simulink model "Adaptive_7DOF"  (R2024a)
settings: Solver=ode4  StartTime=0.0  StopTime=20  FixedStep=0.01  RelTol=1e-3
model workspace (MAT data in the model file):
  e2 = Simulink.Signal
  e2.DataType = 'auto'
  e2.Dimensions = [4 1]
  e2.DimensionsMode = 'Fixed'
  e2.Complexity = 'auto'
  e2.SampleTime = -1
  e2.SamplingMode = 'auto'
libraries: aerolibconvert2 x20
settings Model: Creator=hp  LastModifiedBy=somesh
settings SolverCC: ZeroCrossAlgorithm=Adaptive
settings DataIOCC: ReturnWorkspaceOutputs=off
settings DebuggingCC: IgnoredZcDiagnostic=none  UnderSpecifiedDimensionMsg=warning
settings RTWCC: GPUComputeCapability=3.5

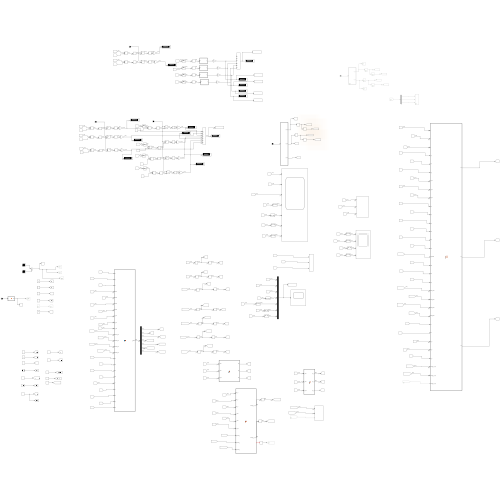
[thumbnail: Simulink's stored preview of the top-level diagram]
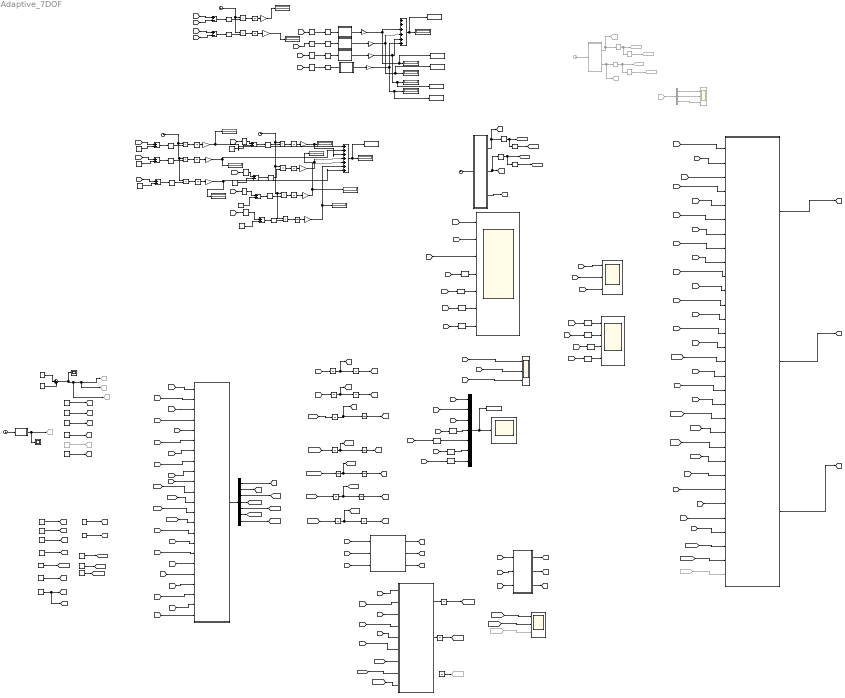
== system Adaptive_7DOF ==
  Abs{,1..12} (13 alike) : Abs  SaturateOnIntegerOverflow=off
  Angle Conversion{,1..19} (20 alike) : aerolibconvert2/Angle Conversion  IU=rad  OU=deg
  Clock{,1,5,7..8} (5 alike) : Clock
  Clock2 : Clock  Commented=on
  Constant : Constant  Value=6.1
  Constant1 : Constant  Value=15.6
  Constant10 : Constant  Value=14.77
  Constant11 : Constant  Value=0.5
  Constant12 : Constant  Value=0.6
  Constant13 : Constant  Value=32.11
  Constant14 : Constant  Value=30
  Constant15 : Constant  Value=17.55
  Constant{3,8,16..17} (4 alike) : Constant
  Constant18 : Constant  Value=29.41
  Constant19 : Constant  Value=43.34
  Constant2 : Constant  Value=2
  Constant20 : Constant  Value=1.5
  Constant21 : Constant  Value=0.01
  Constant22 : Constant  Value=0.005
  Constant4 : Constant  Commented=on  Value=0.5
  Constant{6..7,48..49} (4 alike) : Constant  Value=0
  Constant5 : Constant  Value=0.5
  Constant9 : Constant  Value=0.7
  Demux : Demux  Outputs=7
  Demux3 : Demux  Commented=on  Outputs=3
  Derivative{,1..3} (4 alike) : Derivative
  Derivative{4..7} (4 alike) : Derivative  Commented=on
  Display{1..4,25,28..29,39,53..59} (15 alike) : Display
  From110 : From  Commented=on  GotoTag=omega_z_cap
  From170 : From  Commented=on  GotoTag=qx_d
  From98 : From  Commented=on  GotoTag=omega_z_cap
  Gain{,1..12} (13 alike) : Gain
  Goto18 : Goto  Commented=on  GotoTag=Fx
  Goto19 : Goto  Commented=on  GotoTag=Fy
  Goto24 : Goto  Commented=on  GotoTag=l1
  Goto49 : Goto  Commented=on  GotoTag=qs_d
  Goto51 : Goto  Commented=on  GotoTag=qx_d
  Goto52 : Goto  Commented=on  GotoTag=Fz
  Goto53 : Goto  Commented=on  GotoTag=qs_d_Dot
  Goto54 : Goto  Commented=on  GotoTag=qs_d_DDot
  Goto55 : Goto  Commented=on  GotoTag=qx_d_Dot
  Goto56 : Goto  Commented=on  GotoTag=qx_d_DDot
  Goto61 : Goto  Commented=on  GotoTag=m2
  Goto64 : Goto  Commented=on  GotoTag=omega_z_cap
  Integrator{,1..7,12..20,22..25} (21 alike) : Integrator
  Integrator{8..11} (4 alike) : Integrator  WrapState=on  WrappedStateUpperValue=pi/2  WrappedStateLowerValue=-pi/2
  Integrator21 : Integrator  InitialCondition=0.5
  MATLAB Function : MATLAB Function  TreatAsAtomicUnit=on
  MATLAB Function1 : MATLAB Function  TreatAsAtomicUnit=on
  MATLAB Function13 : MATLAB Function  TreatAsAtomicUnit=on
  MATLAB Function16 : MATLAB Function  TreatAsAtomicUnit=on
  MATLAB Function2 : MATLAB Function  TreatAsAtomicUnit=on
  MATLAB Function20 : MATLAB Function  TreatAsAtomicUnit=on
  MATLAB Function3 : MATLAB Function  TreatAsAtomicUnit=on
  MATLAB Function4 : MATLAB Function  TreatAsAtomicUnit=on
  MATLAB Function5 : MATLAB Function  TreatAsAtomicUnit=on
  MATLAB Function6 : MATLAB Function  Commented=on  TreatAsAtomicUnit=on
  MATLAB Function7 : MATLAB Function  TreatAsAtomicUnit=on
  MATLAB Function8 : MATLAB Function  TreatAsAtomicUnit=on
  Mux12 : Mux  Inputs=7
  Product{,1..8} (9 alike) : Product
  Pulse Generator : DiscretePulseGenerator  PulseType=Time based  Amplitude=20  Period=100  PhaseDelay=1
  Pulse Generator1 : DiscretePulseGenerator  PulseType=Time based  Amplitude=-20  Period=100  PhaseDelay=2
  Scope : Scope  NumInputPorts=7
  Scope1 : Scope
  Scope13 : Scope
  Scope2 : Scope
  Scope3 : Scope  NumInputPorts=3
  Scope4 : Scope  NumInputPorts=3
  Scope5 : Scope  NumInputPorts=3
  Scope6 : Scope  NumInputPorts=4
  Scope9 : Scope  Commented=on  NumInputPorts=3
  Subtract{1..5,16..17,19..20} (9 alike) : Sum  Inputs=+-
  Sum : Sum  Inputs=|+++++++
  Sum2 : Sum  Inputs=|++
  Sum4 : Sum  Inputs=|++++++
  To Workspace : ToWorkspace  VariableName=theta_m  SampleTime=-1
  To Workspace1 : ToWorkspace  VariableName=ITAE  SampleTime=-1
  To Workspace2 : ToWorkspace  VariableName=theta_m1  SampleTime=-1
  To Workspace20 : ToWorkspace  VariableName=values  SaveFormat=Timeseries  SampleTime=-1
  To Workspace3 : ToWorkspace  VariableName=theta_m2  SampleTime=-1
  To Workspace4 : ToWorkspace  VariableName=theta_m3  SampleTime=-1
  To Workspace5 : ToWorkspace  VariableName=theta_m4  SampleTime=-1
  wires:
  [x_ddot] -> Integrator/1
  Integrator/1 -> Integrator6/1, [x_dot]
  [y_ddot] -> Integrator1/1
  Integrator1/1 -> Integrator7/1, [y_dot]
  [theta1_ddot] -> Integrator2/1
  Integrator2/1 -> Integrator8/1, [theta1_dot]
  [theta2_ddot] -> Integrator3/1
  Integrator3/1 -> Integrator9/1, [theta2_dot]
  [theta3_ddot] -> Integrator4/1
  Integrator4/1 -> Integrator10/1, [theta3_dot]
  [theta4_ddot] -> Integrator5/1
  Integrator5/1 -> Integrator11/1, [theta4_dot]
  Integrator6/1 -> [x]
  Integrator7/1 -> [y]
  Integrator8/1 -> [theta1]
  Integrator9/1 -> [theta2]
  Integrator10/1 -> [theta3]
  Integrator11/1 -> [theta4]
  [theta1] -> MATLAB Function/4(theta1)
  [theta2] -> MATLAB Function/5(theta2)
  [theta3] -> MATLAB Function/6(theta3)
  [theta4] -> MATLAB Function/7(theta4)
  [theta1_dot] -> MATLAB Function/11(theta1_dot)
  [theta2_dot] -> MATLAB Function/12(theta2_dot)
  [theta3_dot] -> MATLAB Function/13(theta3_dot)
  [theta4_dot] -> MATLAB Function/14(theta4_dot)
  Pulse Generator1/1 -> Sum2/2
  Pulse Generator/1 -> Sum2/1
  Sum2/1 -> Scope1/1, Goto52/1, Goto19/1, Goto18/1
  [m1] -> MATLAB Function/15(m1)
  [m2] -> MATLAB Function/16(m2)
  [M1] -> MATLAB Function/17(M1)
  [M2] -> MATLAB Function/18(M2)
  [l1] -> MATLAB Function/19(l1)
  [l2] -> MATLAB Function/20(l2)
  Constant/1 -> [M1]
  Constant1/1 -> [M2]
  Constant2/1 -> [m1]
  Constant3/1 -> [m2]
  Constant4/1 -> Goto24/1
  Constant5/1 -> [l2]
  Subtract16/1 -> Abs/1
  Integrator13/1 -> Gain3/1
  Constant7/1 -> Subtract20/2
  Gain2/1 -> Sum/3, Display39/1
  Integrator15/1 -> Gain5/1
  Gain1/1 -> Display25/1, Sum/2
  Product1/1 -> Integrator17/1
  Abs/1 -> Product/2
  [y] -> Subtract17/1
  Product2/1 -> Integrator14/1
  Subtract20/1 -> Abs4/1
  Abs2/1 -> Product2/2
  Abs3/1 -> Product3/2
  Gain5/1 -> Sum/6, Display29/1
  Abs5/1 -> Product5/2
  Integrator17/1 -> Gain1/1
  Clock8/1 -> Product5/1, Product2/1, Product4/1, Product3/1
  Gain3/1 -> Display1/1, Sum/4
  Subtract1/1 -> Abs2/1
  Constant48/1 -> Subtract1/2
  Integrator16/1 -> Gain/1
  Gain/1 -> Sum/1, Display3/1
  Product4/1 -> Integrator13/1
  Integrator14/1 -> Gain4/1
  Constant6/1 -> Subtract19/2
  Integrator12/1 -> Gain2/1
  Constant12/1 -> Subtract17/2
  Product5/1 -> Integrator15/1
  Subtract2/1 -> Abs5/1
  Abs4/1 -> Product4/2
  Product/1 -> Integrator16/1
  Gain4/1 -> Display28/1, Sum/5
  [x] -> Subtract16/1
  Constant49/1 -> Subtract2/2
  Subtract17/1 -> Abs1/1
  Constant11/1 -> Subtract16/2
  Sum/1 -> Display4/1, To Workspace1/1
  Product3/1 -> Integrator12/1
  Abs1/1 -> Product1/2
  [theta2] -> Angle Conversion9/1
  Gain11/1 -> Sum4/6, To Workspace5/1, Display56/1
  Subtract4/1 -> Abs7/1
  Gain10/1 -> To Workspace4/1, Display58/1, Sum4/5
  Subtract3/1 -> Abs6/1
  Abs11/1 -> MATLAB Function2/1(u)
  MATLAB Function20/1(y) -> Gain11/1
  [x_d] -> Subtract3/2
  [y_d] -> Subtract4/2
  [x] -> Subtract3/1
  MATLAB Function2/1(y) -> Gain8/1
  [theta4] -> Angle Conversion11/1
  Clock5/1 -> Product7/1, Product6/1
  MATLAB Function16/1(y) -> Gain10/1
  [theta3] -> Angle Conversion10/1
  Abs6/1 -> Product6/2
  [y] -> Subtract4/1
  Abs9/1 -> MATLAB Function16/1(u)
  Integrator18/1 -> Gain6/1
  Sum4/1 -> To Workspace/1, Display59/1
  Abs10/1 -> MATLAB Function20/1(u)
  MATLAB Function13/1(y) -> Gain9/1
  Product7/1 -> Integrator19/1
  Abs8/1 -> MATLAB Function13/1(u)
  [theta1] -> Angle Conversion8/1
  Gain7/1 -> Display54/1
  Product6/1 -> Integrator18/1
  Gain6/1 -> Display57/1
  Abs7/1 -> Product7/2
  Gain9/1 -> Sum4/4, To Workspace3/1, Display55/1
  Integrator19/1 -> Gain7/1
  Subtract19/1 -> Abs3/1
  [theta1] -> Angle Conversion4/1
  Angle Conversion4/1 -> Subtract19/1
  [theta2] -> Angle Conversion5/1
  Angle Conversion5/1 -> Subtract20/1
  [theta3] -> Angle Conversion6/1
  Angle Conversion6/1 -> Subtract1/1
  [theta4] -> Angle Conversion7/1
  Angle Conversion7/1 -> Subtract2/1
  Angle Conversion8/1 -> Abs11/1
  Angle Conversion9/1 -> Abs8/1
  Angle Conversion10/1 -> Abs9/1
  Angle Conversion11/1 -> Abs10/1
  [theta3] -> Angle Conversion16/1
  [theta1] -> Angle Conversion14/1
  Mux12/1 -> Scope2/1, To Workspace20/1
  [theta2] -> Angle Conversion15/1
  [theta4] -> Angle Conversion17/1
  [x] -> Scope/1
  [y] -> Scope/2
  [theta4] -> Angle Conversion3/1
  [theta3] -> Angle Conversion2/1
  [theta1] -> Angle Conversion/1
  [theta2] -> Angle Conversion1/1
  [Fx] -> MATLAB Function/1(Fx)
  [Fy] -> MATLAB Function/2(Fy)
  MATLAB Function/1(q_ddot) -> Demux/1
  [x_dot] -> MATLAB Function/8(x_dot)
  [y_dot] -> MATLAB Function/9(y_dot)
  Gain8/1 -> To Workspace2/1, Display53/1, Sum4/3
  [Fx] -> Scope3/1
  [Fy] -> Scope3/2
  MATLAB Function4/1(m2) -> Goto61/1, Scope13/1
  Clock1/1 -> MATLAB Function4/1(t)
  [x_dot] -> MATLAB Function7/1(x_dot)
  [y_dot] -> MATLAB Function7/2(y_dot)
  MATLAB Function7/1(Frx) -> [Frx]
  MATLAB Function7/2(Fry) -> [Fry]
  [Frx] -> MATLAB Function/21(Frx)
  [Fry] -> MATLAB Function/22(Fry)
  [Fz] -> MATLAB Function/3(Fz)
  [l1_dot] -> MATLAB Function7/3(l1_dot)
  MATLAB Function7/3(Frz) -> [Frz]
  Demux/7 -> [theta4_ddot]
  Demux/6 -> [theta3_ddot]
  Demux/5 -> [theta2_ddot]
  Demux/4 -> [theta1_ddot]
  Demux/2 -> [y_ddot]
  Demux/1 -> [x_ddot]
  [l1_dot] -> MATLAB Function/10(l1_dot)
  [Frz] -> MATLAB Function/23(Frz)
  [l1_ddot] -> Integrator20/1
  Integrator20/1 -> [l1_dot], Integrator21/1
  Integrator21/1 -> [l1]
  [Fz] -> Scope3/3
  [x] -> Mux12/1
  [y] -> Mux12/2
  [l1] -> Mux12/3
  Angle Conversion14/1 -> Mux12/4
  Angle Conversion15/1 -> Mux12/5
  Angle Conversion16/1 -> Mux12/6
  Angle Conversion17/1 -> Mux12/7
  [l1] -> Scope/3
  Angle Conversion/1 -> Scope/4
  Angle Conversion1/1 -> Scope/5
  Angle Conversion2/1 -> Scope/6
  Angle Conversion3/1 -> Scope/7
  Demux/3 -> [l1_ddot]
  Abs12/1 -> Product8/2
  Subtract5/1 -> Abs12/1
  Constant9/1 -> Subtract5/2
  Clock7/1 -> Product8/1, Product1/1, Product/1
  Integrator22/1 -> Gain12/1
  [l1] -> Subtract5/1
  Product8/1 -> Integrator22/1
  Gain12/1 -> Sum/7, Display2/1
  [y_dot] -> MATLAB Function3/8(y_dot)
  [x_dot] -> MATLAB Function3/7(x_dot)
  MATLAB Function3/2(Fy) -> [Fy]
  MATLAB Function3/1(Fx) -> [Fx]
  [x] -> MATLAB Function3/1(x)
  [y] -> MATLAB Function3/2(y)
  [x_d] -> MATLAB Function3/4(x_d)
  [y_d] -> MATLAB Function3/5(y_d)
  [kpx] -> MATLAB Function3/10(kpx)
  [kpy] -> MATLAB Function3/11(kpy)
  [kdx] -> MATLAB Function3/13(kdx)
  [kdy] -> MATLAB Function3/14(kdy)
  [k_lambda] -> MATLAB Function3/16(k_lambda)
  [zeta] -> MATLAB Function3/17(zeta)
  [kwx] -> MATLAB Function3/18(kwx)
  [kwy] -> MATLAB Function3/19(kwy)
  [theta1_dot] -> MATLAB Function3/20(theta1_dot)
  [theta2_dot] -> MATLAB Function3/21(theta2_dot)
  [theta3_dot] -> MATLAB Function3/22(theta3_dot)
  [theta4_dot] -> MATLAB Function3/23(theta4_dot)
  Constant22/1 -> [zeta]
  Constant21/1 -> [k_lambda]
  Constant20/1 -> [kwx], [kwy]
  Constant19/1 -> [kdy]
  Constant10/1 -> [kpx]
  Constant14/1 -> [kpy]
  Constant18/1 -> [kdx]
  MATLAB Function5/2(py_d) -> Derivative2/1, [y_d]
  Derivative1/1 -> [x_d_DDot]
  MATLAB Function5/1(px_d) -> [x_d], Derivative/1
  Derivative/1 -> [x_d_Dot], Derivative1/1
  Clock/1 -> MATLAB Function5/1(t)
  Derivative2/1 -> [y_d_Dot], Derivative3/1
  Derivative3/1 -> [y_d_DDot]
  MATLAB Function3/3(Fz) -> [Fz]
  [l1] -> MATLAB Function3/3(l1)
  [l1_d] -> MATLAB Function3/6(l1_d)
  [l1_dot] -> MATLAB Function3/9(l1_dot)
  [kpz] -> MATLAB Function3/12(kpz)
  [kdz] -> MATLAB Function3/15(kdz)
  [m1] -> MATLAB Function3/24(m1)
  [m2] -> MATLAB Function3/25(m2)
  Constant13/1 -> [kpz]
  Constant15/1 -> [kdz]
  MATLAB Function5/3(pz_d) -> [l1_d]
  [x] -> Scope4/1
  [y] -> Scope4/2
  [theta2] -> Angle Conversion13/1
  [theta3] -> Angle Conversion18/1
  Angle Conversion18/1 -> Scope6/3
  Angle Conversion19/1 -> Scope6/4
  Angle Conversion13/1 -> Scope6/2
  [l1] -> Scope4/3
  Angle Conversion12/1 -> Scope6/1
  [theta1] -> Angle Conversion12/1
  [theta4] -> Angle Conversion19/1
  Demux3/3 -> Scope9/3
  From170/1 -> Demux3/1
  Derivative5/1 -> Goto54/1
  Derivative6/1 -> Derivative7/1, Goto55/1
  MATLAB Function6/1(qs_d) -> Derivative4/1, Goto49/1
  Demux3/1 -> Scope9/1
  Demux3/2 -> Scope9/2
  Clock2/1 -> MATLAB Function6/1(t)
  Derivative4/1 -> Derivative5/1, Goto53/1
  Derivative7/1 -> Goto56/1
  MATLAB Function6/2(qx_d) -> Goto51/1, Derivative6/1
  [phi_x] -> MATLAB Function3/26(phi_x)
  [omega_x_cap] -> MATLAB Function3/29(omega_x_cap)
  [omega_y_cap] -> MATLAB Function3/30(omega_y_cap)
  From98/1 -> MATLAB Function3/31(omega_z_cap)
  [phi_y] -> MATLAB Function3/27(phi_y)
  [phi_z] -> MATLAB Function3/28(phi_z)
  [x_dot] -> MATLAB Function1/1(x_dot)
  [y_dot] -> MATLAB Function1/2(y_dot)
  [l1_dot] -> MATLAB Function1/3(l1_dot)
  MATLAB Function1/1(phi_x) -> [phi_x]
  MATLAB Function1/2(phi_y) -> [phi_y]
  MATLAB Function1/3(phi_z) -> [phi_z]
  MATLAB Function8/1(omega_x_cap) -> Integrator23/1
  ? -> Integrator25/1
  MATLAB Function8/2(omega_y_cap) -> Integrator24/1
  [phi_x] -> MATLAB Function8/1(phi_x)
  [phi_x] -> MATLAB Function8/2(phi_y)
  [phi_x] -> MATLAB Function8/3(phi_z)
  [x_dot] -> MATLAB Function8/4(x_dot)
  [y_dot] -> MATLAB Function8/5(y_dot)
  [l1_dot] -> MATLAB Function8/6(l1_dot)
  Integrator23/1 -> [omega_x_cap]
  Integrator24/1 -> [omega_y_cap]
  Integrator25/1 -> Goto64/1
  [omega_x_cap] -> Scope5/1
  [omega_y_cap] -> Scope5/2
  From110/1 -> Scope5/3
  [gamma_x] -> MATLAB Function8/7(gamma_x)
  [gamma_y] -> MATLAB Function8/8(gamma_y)
  [gamma_z] -> MATLAB Function8/9(gamma_z)
  Constant17/1 -> [gamma_z]
  Constant16/1 -> [gamma_y]
  Constant8/1 -> [gamma_x]

== matlab function Adaptive_7DOF/MATLAB Function8 ==
  data: phi_x input; omega_x_cap output; phi_y input; phi_z input; x_dot input; y_dot input; l1_dot input; omega_y_cap output; gamma_x input; gamma_y input; gamma_z input
function [omega_x_cap, omega_y_cap] = fcn(phi_x, phi_y, phi_z, x_dot, y_dot, l1_dot,gamma_x,gamma_y,gamma_z)

omega_x_cap = -gamma_x*phi_x*x_dot;
omega_y_cap = -gamma_y*phi_y*y_dot;
% omega_z_cap = -gamma_z*phi_z*l1_dot;
end

== matlab function Adaptive_7DOF/MATLAB Function3 ==
  data: x input; Fx output; y input; l1 input; x_d input; y_d input; l1_d input; x_dot input; y_dot input; l1_dot input; kpx input; kpy input; kpz input; kdx input; kdy input; kdz input; k_lambda input; zeta input; kwx input; kwy input; theta1_dot input; theta2_dot input; theta3_dot input; theta4_dot input; m1 input; m2 input; Fy output; phi_x input; phi_y input; Fz output; phi_z input size=[1 1]; omega_x_cap input; omega_y_cap input; omega_z_cap input size=[1 1]
function [Fx, Fy, Fz] = fcn(x, y, l1, x_d, y_d, l1_d, x_dot, y_dot, l1_dot, kpx, kpy, kpz, kdx, kdy, kdz, k_lambda, zeta, kwx, kwy,...
    theta1_dot, theta2_dot, theta3_dot, theta4_dot, m1, m2, phi_x, phi_y, phi_z, omega_x_cap, omega_y_cap, omega_z_cap)

g=9.8;
ex = x-x_d;
ey = y-y_d;
ez = l1 - l1_d;

% Fx = -kpx*ex - kdx*x_dot - k_lambda*((x_d + zeta)^2 - x^2 + ex*x/((x_d + zeta)^2 - x^2)^2)*ex + phi_x*omega_x_cap - kwx*(theta1_dot^2 + theta2_dot^2 + theta3_dot^2 + theta4_dot^2)*x_dot;
% 
% Fy = -kpy*ey - kdy*y_dot - k_lambda*((y_d + zeta)^2 - y^2 + ey*y/((y_d + zeta)^2 - y^2)^2)*ey + phi_y*omega_y_cap - kwy*(theta1_dot^2 + theta2_dot^2 + theta3_dot^2 + theta4_dot^2)*y_dot;


Fx = -kpx*ex - kdx*x_dot - k_lambda*(((x_d + zeta)^2 - x^2 + ex*x)/(((x_d + zeta)^2 - x^2)^2))*ex  - kwx*(theta1_dot^2 + theta2_dot^2 + theta3_dot^2 + theta4_dot^2)*x_dot + phi_x'*omega_x_cap;

Fy = -kpy*ey - kdy*y_dot - k_lambda*(((y_d + zeta)^2 - y^2 + ey*y)/(((y_d + zeta)^2 - y^2)^2))*ey  - kwy*(theta1_dot^2 + theta2_dot^2 + theta3_dot^2 + theta4_dot^2)*y_dot + phi_y'*omega_y_cap;

Fz = -kpz*ez - kdz*l1_dot - k_lambda*(((l1_d + zeta)^2 - l1^2 + ez*l1)/(((l1_d + zeta)^2 - l1^2)^2))*ez  - (m1 + m2)*g ;

end

== matlab function Adaptive_7DOF/MATLAB Function6 ==
  data: t input; qs_d output; qx_d output
function [qs_d, qx_d] = fcn(t)

qs_d = zeros(4,1);
qx_d = [0;0; 0];

x0=0;
y0=0;
z0=0;
x_d=0.5;
y_d=0.6;
z_d=0.7;
kv= 0.4;
ka = 0.4;
epsilon = 1.5;
k1 = (2*ka)/kv;
k2 = (2*ka)/(kv^2);
qx_d(1) = x0 + (x_d/2) + (kv/(2*k1))*(sqrt(1+(k1*t - epsilon)^2) - sqrt(1 + (k1*t - epsilon - k2*x_d)^2));
qx_d(2) = y0 + (y_d/2) + (kv/(2*k1))*(sqrt(1+(k1*t - epsilon)^2) - sqrt(1 + (k1*t - epsilon - k2*y_d)^2));
qx_d(3) = z0 + (z_d/2) + (kv/(2*k1))*(sqrt(1+(k1*t - epsilon)^2) - sqrt(1 + (k1*t - epsilon - k2*z_d)^2));

end


% if t >= 0 && t <= 20
%     
%   x_d = 0.02*t^2;
%   y_d = 0.03*t^2 ;
% 
%   
% elseif t >= 20 && t <= 60
%     
%   x_d = 8;
%   y_d = 12;
% 
%   
% elseif t >= 60 && t <= 80
%     
%   x_d = 8 + ((t - (60))^2)*0.03;
%   y_d = 12 + ((t-(60))^2)*0.02;
% 
%   
% else
%     x_d = 20;
%     y_d = 20;

== matlab function Adaptive_7DOF/MATLAB Function16 ==
  settings: updateMethod=DISCRETE
  data: u input; y output
function y = fcn(u)
    persistent maxVal;
    
    % Check if maxVal is empty and initialize it if necessary
    if isempty(maxVal)
        maxVal = 0; % Initialize with negative infinity or another suitable value
    end
    
    % Update maxVal if the current input is greater
    if u > maxVal
        maxVal = u;
    end
    
    y = maxVal;
end

== matlab function Adaptive_7DOF/MATLAB Function4 ==
  data: t input; m2 output
function m2 = fcn(t)

if t>=0 && t<3
    m2 = 0.6;
else
    m2 = 0.2;

% m2 = 0.6;


end

== matlab function Adaptive_7DOF/MATLAB Function7 ==
  data: x_dot input; Frx output; y_dot input; Fry output; l1_dot input; Frz output
function [Frx, Fry, Frz] = fcn(x_dot, y_dot, l1_dot)

frox = 0.6;
froy = 0.6;
epsilon_x = 0.6;
epsilon_y = 0.6;
krx = 0.1;
kry = 0.1;
dz = 0.1;

Frx = frox*tanh(x_dot/epsilon_x) - krx*abs(x_dot)*x_dot;
Fry = froy*tanh(y_dot/epsilon_y) - kry*abs(y_dot)*y_dot;
Frz = dz * l1_dot;
end

== matlab function Adaptive_7DOF/MATLAB Function2 ==
  settings: updateMethod=DISCRETE
  data: u input; y output
function y = fcn(u)
    persistent maxVal;
    
    % Check if maxVal is empty and initialize it if necessary
    if isempty(maxVal)
        maxVal = 0; % Initialize with negative infinity or another suitable value
    end
    
    % Update maxVal if the current input is greater
    if u > maxVal
        maxVal = u;
    end
    
    y = maxVal;
end

== matlab function Adaptive_7DOF/MATLAB Function20 ==
  settings: updateMethod=DISCRETE
  data: u input; y output
function y = fcn(u)
    persistent maxVal;
    
    % Check if maxVal is empty and initialize it if necessary
    if isempty(maxVal)
        maxVal = 0; % Initialize with negative infinity or another suitable value
    end
    
    % Update maxVal if the current input is greater
    if u > maxVal
        maxVal = u;
    end
    
    y = maxVal;
end

== matlab function Adaptive_7DOF/MATLAB Function1 ==
  data: x_dot input; phi_x output; y_dot input; phi_y output; phi_z output; l1_dot input
function [phi_x, phi_y, phi_z] = fcn(x_dot,y_dot, l1_dot)


epsilon_x = 0.6;
epsilon_y = 0.6;

phi_x = [tanh(x_dot/epsilon_x); abs(x_dot)*x_dot];
phi_y = [tanh(y_dot/epsilon_y); abs(y_dot)*y_dot];
phi_z = l1_dot;

end

== matlab function Adaptive_7DOF/MATLAB Function ==
  data: Fx input size=[1 1]; Fy input size=[1 1]; Fz input size=[1 1]; theta1 input; theta2 input; theta3 input; theta4 input; x_dot input; y_dot input; l1_dot input; theta1_dot input; theta2_dot input; theta3_dot input; theta4_dot input; m1 input; m2 input; M1 input; M2 input; l1 input; l2 input; q_ddot output size=[7 1]; Frx input; Fry input; Frz input
function q_ddot   = fcn(Fx, Fy, Fz, theta1, theta2, theta3, theta4,...
    x_dot, y_dot, l1_dot, theta1_dot, theta2_dot, theta3_dot, theta4_dot,...
    m1, m2, M1, M2, l1, l2, Frx, Fry, Frz)

g = 9.8;


% Mass matrix M(q)
M = zeros(7, 7);

% Define M matrix elements
M(1,1) = M1 + m1 + m2;
M(1,2) = 0;
M(1,3) = (m1 + m2) * sin(theta1) * cos(theta2);
M(1,4) = (m1 + m2) * l1 * cos(theta1) * cos(theta2);
M(1,5) = -(m1 + m2) * l1 * sin(theta1) * sin(theta2);
M(1,6) = m2 * l2 * cos(theta3) * cos(theta4);
M(1,7) = -m2 * l2 * sin(theta3) * sin(theta4);

M(2,1) = 0;
M(2,2) = M2 + m1 + m2;
M(2,3) = (m1 + m2) * sin(theta2);
M(2,4) = 0;
M(2,5) = (m1 + m2) * l1 * cos(theta2);
M(2,6) = 0;
M(2,7) = m2 * l2 * cos(theta4);

M(3,1) = (m1 + m2) * sin(theta1) * cos(theta2);
M(3,2) = (m1 + m2) * sin(theta2);
M(3,3) = m1 + m2;
M(3,4) = 0;
M(3,5) = 0;
M(3,6) = m2 * l2 * cos(theta2) * cos(theta4) * sin(theta1 - theta3);
M(3,7) = m2 * l2 * (sin(theta2) * cos(theta4) - cos(theta2) * sin(theta4) * cos(theta1 - theta3));

M(4,1) = (m1 + m2) * l1 * cos(theta1) * cos(theta2);
M(4,2) = 0;
M(4,3) = 0;
M(4,4) = (m1 + m2) * l1^2 * cos(theta2)^2;
M(4,5) = 0;
M(4,6) = m2*l1*l2*cos(theta2)*cos(theta4)*cos(theta1-theta3);
M(4,7) = m2*l1*l2*cos(theta2)*sin(theta4)*sin(theta1 - theta3);

M(5,1) = -(m1 + m2) * l1 * sin(theta1) * sin(theta2);
M(5,2) = (m1 + m2) * l1 * cos(theta2);
M(5,3) = 0;
M(5,4) = 0;
M(5,5) = (m1 + m2) * l1^2;
M(5,6) = -m2 * l1 * l2 * sin(theta2) * cos(theta4) * sin(theta1 - theta3);
M(5,7) = m2 * l1 * l2 * (cos(theta2) * cos(theta4) + sin(theta2) * sin(theta4) * cos(theta1 - theta3));

M(6,1) = m2 * l2 * cos(theta3) * cos(theta4);
M(6,2) = 0;
M(6,3) = m2 * l2 * cos(theta2) * cos(theta4) * sin(theta1 - theta3);
M(6,4) = m2*l1*l2*cos(theta2)*cos(theta4)*cos(theta1-theta3);
M(6,5) = -m2 * l1 * l2 * sin(theta2) * cos(theta4) * sin(theta1 - theta3);
M(6,6) = m2 * l2^2 * cos(theta4)^2;
M(6,7) = 0;

M(7,1) = -m2 * l2 * sin(theta3) * sin(theta4);
M(7,2) = m2 * l2 * cos(theta4);
M(7,3) = m2 * l2 * (sin(theta2) * cos(theta4) - cos(theta2) * sin(theta4) * cos(theta1 - theta3));
M(7,4) = m2*l1*l2*cos(theta2)*sin(theta4)*sin(theta1 - theta3);
M(7,5) = m2 * l1 * l2 * (cos(theta2) * cos(theta4) + sin(theta2) * sin(theta4) * cos(theta1 - theta3));
M(7,6) = 0;
M(7,7) = m2 * l2^2;

% Coriolis matrix C(q, dq)
C = zeros(7, 7);

% Define C matrix elements
C(1,3) = (m1 + m2) * (cos(theta1) * cos(theta2) * theta1_dot - sin(theta1) * sin(theta2) * theta2_dot);
C(1,4) = (m1 + m2) * (cos(theta1) * cos(theta2) * l1_dot - l1 * sin(theta1) * sin(theta2) * theta1_dot - l1 * cos(theta1) * sin(theta2) * theta2_dot);
C(1,5) = -(m1 + m2) * (sin(theta1) * sin(theta2) * l1_dot + l1 * cos(theta1) * sin(theta2) * theta1_dot + l1 * sin(theta1) * cos(theta2) * theta2_dot);
C(1,6) = -m2 * l2 * (sin(theta3) * cos(theta4) * theta3_dot + cos(theta3) * sin(theta4) * theta4_dot);
C(1,7) = -m2 * l2 * (cos(theta3) * sin(theta4) * theta3_dot + sin(theta3) * cos(theta4) * theta4_dot);

C(2,3) = (m1 + m2) * cos(theta2) * theta2_dot;
C(2,5) = (m1 + m2) * (cos(theta2) * l1_dot - l1 * sin(theta2) * theta2_dot);
C(2,7) = -m2 * l2 * sin(theta4) * theta4_dot;

C(3,4) = -(m1 + m2) * l1 * cos(theta2)^2 * theta1_dot;
C(3,5) = -(m1 + m2) * l1 * theta2_dot;
C(3,6) = -m2 * l2 * (cos(theta2) * cos(theta4) * cos(theta1 - theta3) * theta3_dot + cos(theta2) * sin(theta4) * sin(theta1 - theta3) * theta4_dot);
C(3,7) = -m2 * l2 * (cos(theta2) * sin(theta4) * theta3_dot + sin(theta2) * sin(theta4) * theta4_dot + cos(theta2) * cos(theta4) * cos(theta1 - theta3) * theta4_dot);

C(4,3) = (m1 + m2) * l1 * cos(theta2)^2 * theta1_dot;
C(4,4) = (m1 + m2) * (l1 * cos(theta2)^2 * l1_dot - l1^2 * sin(theta2) * cos(theta2) * theta2_dot);
C(4,5) = -(m1 + m2) * l1^2 * sin(theta2) * cos(theta2) * theta1_dot;
C(4,6) = m2 * l1 * l2 * (cos(theta2) * cos(theta4) * sin(theta1 - theta3) * theta3_dot + cos(theta2) * sin(theta4) * cos(theta1 - theta3) * theta4_dot);
C(4,7) = m2 * l1 * l2 * (cos(theta2) * cos(theta4) * sin(theta1 - theta3) * theta4_dot + cos(theta2) * sin(theta4) * cos(theta1 - theta3) * theta3_dot);

C(5,3) = (m1 + m2) * l1 * theta2_dot;
C(5,4) = (m1 + m2) * l1^2 * sin(theta2) * cos(theta2) * theta1_dot;
C(5,5) = (m1 + m2) * l1 * l1_dot;
C(5,6) = m2 * l1 * l2 * (sin(theta2) * cos(theta4) * cos(theta1 - theta3) * theta3_dot + sin(theta2) * sin(theta4) * sin(theta1 - theta3) * theta4_dot);
C(5,7) = m2 * l1 * l2 * (sin(theta2) * sin(theta4) * sin(theta1 - theta3) * theta3_dot + sin(theta2) * cos(theta4) * cos(theta1 - theta3) * theta4_dot ...
    - cos(theta2) * sin(theta4) * theta4_dot);

C(6,3) = m2 * l2 * (cos(theta2) * cos(theta4) * cos(theta1 - theta3) * theta1_dot - sin(theta2) * cos(theta4) * sin(theta1 - theta3) * theta2_dot);
C(6,4) = m2 * l2 * (cos(theta2) * cos(theta4) * cos(theta1 - theta3) * l1_dot - l1 * cos(theta2) * cos(theta4) * sin(theta1 - theta3) ...
    * theta1_dot - l1 * sin(theta2) * cos(theta4) * cos(theta1 - theta3) * theta2_dot);
C(6,5) = -m2 * l2 * (sin(theta2) * cos(theta4) * sin(theta1 - theta3) * l1_dot + l1 * sin(theta2) * cos(theta4) * cos(theta1 - theta3) ...
    * theta1_dot + l1 * cos(theta2) * cos(theta4) * sin(theta1 - theta3) * theta2_dot);
C(6,6) = -m2 * l2^2 * sin(theta4) * cos(theta4) * theta4_dot;
C(6,7) = -m2 * l2^2 * sin(theta4) * cos(theta4) * theta3_dot;

C(7,3) = m2 * l2 * (cos(theta2) * sin(theta4) * sin(theta1 - theta3) * theta1_dot + sin(theta2) * sin(theta4) * cos(theta1 - theta3) * theta2_dot ...
    + cos(theta2) * cos(theta4) * theta2_dot);
C(7,4) = m2 * l2 * (cos(theta2) * sin(theta4) * sin(theta1 - theta3) * l1_dot + l1 * cos(theta2) * sin(theta4) * cos(theta1 - theta3) ...
    * theta1_dot - l1 * sin(theta2) * sin(theta4) * sin(theta1 - theta3)*theta2_dot);
C(7,5) = m2 * l2 * (cos(theta2)*cos(theta4)*l1_dot + sin(theta2)*sin(theta4)*cos(theta1 - theta3)*l1_dot - l1 * sin(theta2)*sin(theta4)...
    *sin(theta1 - theta3)*theta1_dot + l1*cos(theta2)*sin(theta4)*cos(theta1 - theta3)*theta2_dot - l1*sin(theta2)*cos(theta4)*theta2_dot);
C(7,6) = m2 * l2^2 * sin(theta4) * cos(theta4) * theta3_dot;

% Gravity with friction matrix
G = zeros(7, 1);

% Define G matrix elements
G(1,1) = Frx;
G(2,1) = Fry;
G(3,1) = Frz - (m1 + m2) * g * cos(theta1) * cos(theta2);
% G(3,1) = 0;
G(4,1) = (m1 + m2) * g * l1 * sin(theta1) * cos(theta2);
G(5,1) = (m1 + m2) * g * l1 * cos(theta1) * sin(theta2);
G(6,1) = m2 * g * l2 * sin(theta3) * cos(theta4);
G(7,1) = m2 * g * l2 * cos(theta3) * sin(theta4);


q_dot = [x_dot; y_dot; l1_dot; theta1_dot; theta2_dot; theta3_dot; theta4_dot];
tau = [Fx; Fy; Fz; 0; 0; 0; 0];
D = tau - C*q_dot - G;

q_ddot = M\D;

end

== matlab function Adaptive_7DOF/MATLAB Function13 ==
  settings: updateMethod=DISCRETE
  data: u input; y output
function y = fcn(u)
    persistent maxVal;
    
    % Check if maxVal is empty and initialize it if necessary
    if isempty(maxVal)
        maxVal = 0; % Initialize with negative infinity or another suitable value
    end
    
    % Update maxVal if the current input is greater
    if u > maxVal
        maxVal = u;
    end
    
    y = maxVal;
end

== matlab function Adaptive_7DOF/MATLAB Function5 ==
  data: t input; px_d output; py_d output; pz_d output
function [px_d, py_d, pz_d] = fcn(t)
% x_d = 0.5;
% y_d = 0.6;
% l1_d = 0.7;

x0=0;
y0=0;
z0=0.5;
x_d=0.5;
y_d=0.6;
z_d=0.2;
kv= 0.4;
ka = 0.4;
epsilon = 1.5;
k1 = (2*ka)/kv;
k2 = (2*ka)/(kv^2);
px_d = x0 + (x_d/2) + (kv/(2*k1))*(sqrt(1+(k1*t - epsilon)^2) - sqrt(1 + (k1*t - epsilon - k2*x_d)^2));
py_d = y0 + (y_d/2) + (kv/(2*k1))*(sqrt(1+(k1*t - epsilon)^2) - sqrt(1 + (k1*t - epsilon - k2*y_d)^2));
pz_d = z0 + (z_d/2) + (kv/(2*k1))*(sqrt(1+(k1*t - epsilon)^2) - sqrt(1 + (k1*t - epsilon - k2*z_d)^2));


end

% function [qs_d, qx_d] = fcn(t)
% 
% qs_d = zeros(4,1);
% qx_d = [0;0; 0];
% 
% x0=0;
% y0=0;
% z0=0;
% x_d=0.5;
% y_d=0.6;
% z_d=0.7;
% kv= 0.4;
% ka = 0.4;
% epsilon = 1.5;
% k1 = (2*ka)/kv;
% k2 = (2*ka)/(kv^2);
% qx_d(1) = x0 + (x_d/2) + (kv/(2*k1))*(sqrt(1+(k1*t - epsilon)^2) - sqrt(1 + (k1*t - epsilon - k2*x_d)^2));
% qx_d(2) = y0 + (y_d/2) + (kv/(2*k1))*(sqrt(1+(k1*t - epsilon)^2) - sqrt(1 + (k1*t - epsilon - k2*y_d)^2));
% qx_d(3) = z0 + (z_d/2) + (kv/(2*k1))*(sqrt(1+(k1*t - epsilon)^2) - sqrt(1 + (k1*t - epsilon - k2*z_d)^2));
% 
% end


% if t >= 0 && t <= 20
%     
%   x_d = 0.02*t^2;
%   y_d = 0.03*t^2 ;
% 
%   
% elseif t >= 20 && t <= 60
%     
%   x_d = 8;
%   y_d = 12;
% 
%   
% elseif t >= 60 && t <= 80
%     
%   x_d = 8 + ((t - (60))^2)*0.03;
%   y_d = 12 + ((t-(60))^2)*0.02;
% 
%   
% else
%     x_d = 20;
%     y_d = 20;
    


% if t>=0 && t<15
%     x_d = 0.2;
%     y_d = 0.6;
% elseif t>=15 && t<20
%     x_d = 0.5;
%     y_d = 0.6;
% else
%     x_d = 0.5;
%     y_d = 0.3;
% end
% end

% if t>=0 && t<15
%     qx_d = [0.2; 0.6];
% elseif t>=15 && t<20
%     qx_d = [0.5; 0.6];
% else
%     qx_d = [0.5; 0.3];
% 
% end


% if t >= 0 && t <= 20
%     
%   x_d = 0.02*t^2;
%   y_d = 0.03*t^2 ;
% 
%   
% elseif t >= 20 && t <= 60
%     
%   x_d = 8;
%   y_d = 12;
% 
%   
% elseif t >= 60 && t <= 80
%     
%   x_d = 8 + ((t - (60))^2)*0.03;
%   y_d = 12 + ((t-(60))^2)*0.02;
% 
%   
% else
%     x_d = 20;
%     y_d = 20;
